simulink subsystem "Simple_Spring_and_Damper_Suspension2"  (R2025b)
settings: Solver=VariableStepAuto  StartTime=0.0  StopTime=10.0  RelTol=1e-3
undefined symbols (not defined in the file): MotoRearSuspDamp, MotoRearSuspEqlbrmLngth, MotoRearSuspStf
settings Model: Creator=The MathWorks, Inc.  LastModifiedBy=The MathWorks, Inc.
settings RTWCC: GPUComputeCapability=3.5

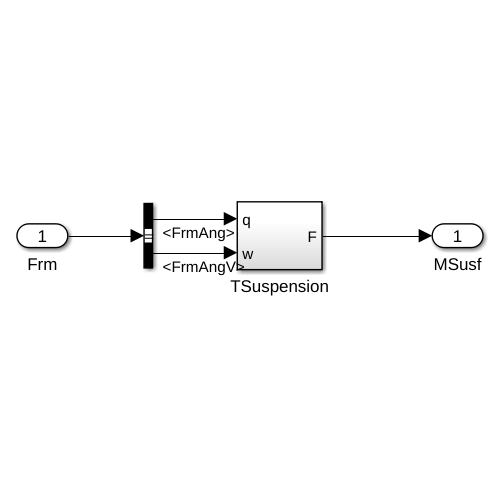
[thumbnail: Simulink's stored preview of the top-level diagram]
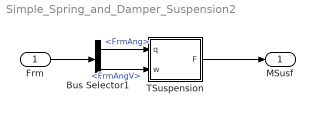
== system Simple_Spring_and_Damper_Suspension2 ==
  Frm : Inport
  Bus Selector1 : BusSelector  OutputSignals=FrmAng,FrmAngV
  TSuspension : Subsystem
  MSusf : Outport
  wires:
  TSuspension/1(F) -> MSusf/1
  Bus Selector1/2 -> TSuspension/2(w)  "<FrmAngV>"
  Bus Selector1/1 -> TSuspension/1(q)  "<FrmAng>"
  Frm/1 -> Bus Selector1/1

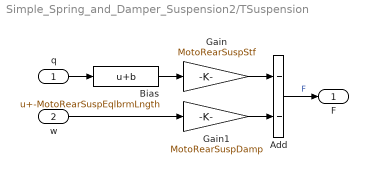
== system Simple_Spring_and_Damper_Suspension2/TSuspension ==
  q : Inport
  w : Inport  Port=2
  Add : Sum  Inputs=--
  Bias : Bias  Bias=-MotoRearSuspEqlbrmLngth  SaturateOnIntegerOverflow=off
  Gain : Gain  Gain=MotoRearSuspStf
  Gain1 : Gain  Gain=MotoRearSuspDamp
  F : Outport
  wires:
  Bias/1 -> Gain/1
  Add/1 -> F/1  "F"
  Gain/1 -> Add/1
  Gain1/1 -> Add/2
  w/1 -> Gain1/1
  q/1 -> Bias/1
